simulink model "oms"  (Simulink 6.5)
settings: Solver=ode45  StartTime=0.0  StopTime=10.0  RelTol=1e-3
libraries: cdsFilt x32, cdsEpicsOut x11, cdsMatrix x4, dac x1, simulink x1, cdsSwitch x1, cdsWD x1, cdsParameters x1
(part 2 of 2)

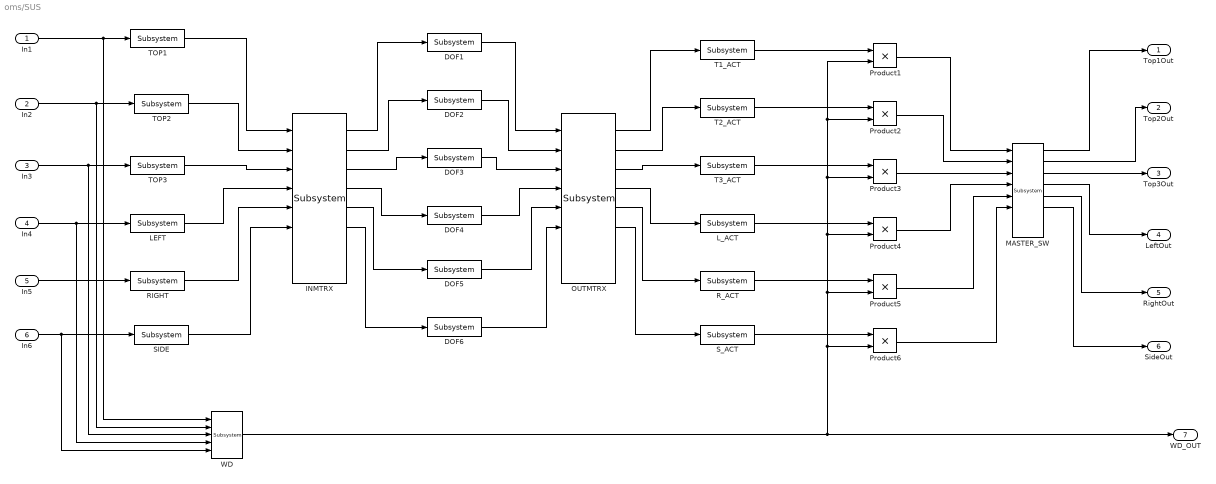
== system oms/SUS ==
  In1 : Inport
  In2 : Inport  Port=2
  In3 : Inport  Port=3
  In4 : Inport  Port=4
  In5 : Inport  Port=5
  In6 : Inport  Port=6
  DOF1 : cdsFilt/Subsystem  Tag=cdsFilt  Description=|  SystemSampleTime=-1
      | Purpose:                                                                                                                                                                                                                                  
      | Standard CDS IIR filter module.                                                                                                                                                                                                           
      |                                                                                                                                                                                                                                           
      | Operation:                                                                                                                                                                                                                                
      | Consists of 10 second order section IIR filters, plus a ramped gain stage. In FE code, also provides pre-defined test points and excitation channel inputs. The filter coefficients are defined in the LIGO system using the 'foton' tool.
      |                                                                                                                                                                                                                                           
      | Usage:                                                                                                                                                                                                                                    
      | Name the part with the desired filter module name.
      settings: AttributesFormatString=%<Tag>
  DOF2 : cdsFilt/Subsystem  Tag=cdsFilt  Description=|  SystemSampleTime=-1
      | Purpose:                                                                                                                                                                                                                                  
      | Standard CDS IIR filter module.                                                                                                                                                                                                           
      |                                                                                                                                                                                                                                           
      | Operation:                                                                                                                                                                                                                                
      | Consists of 10 second order section IIR filters, plus a ramped gain stage. In FE code, also provides pre-defined test points and excitation channel inputs. The filter coefficients are defined in the LIGO system using the 'foton' tool.
      |                                                                                                                                                                                                                                           
      | Usage:                                                                                                                                                                                                                                    
      | Name the part with the desired filter module name.
      settings: AttributesFormatString=%<Tag>
  DOF3 : cdsFilt/Subsystem  Tag=cdsFilt  Description=|  SystemSampleTime=-1
      | Purpose:                                                                                                                                                                                                                                  
      | Standard CDS IIR filter module.                                                                                                                                                                                                           
      |                                                                                                                                                                                                                                           
      | Operation:                                                                                                                                                                                                                                
      | Consists of 10 second order section IIR filters, plus a ramped gain stage. In FE code, also provides pre-defined test points and excitation channel inputs. The filter coefficients are defined in the LIGO system using the 'foton' tool.
      |                                                                                                                                                                                                                                           
      | Usage:                                                                                                                                                                                                                                    
      | Name the part with the desired filter module name.
      settings: AttributesFormatString=%<Tag>
  DOF4 : cdsFilt/Subsystem  Tag=cdsFilt  Description=|  SystemSampleTime=-1
      | Purpose:                                                                                                                                                                                                                                  
      | Standard CDS IIR filter module.                                                                                                                                                                                                           
      |                                                                                                                                                                                                                                           
      | Operation:                                                                                                                                                                                                                                
      | Consists of 10 second order section IIR filters, plus a ramped gain stage. In FE code, also provides pre-defined test points and excitation channel inputs. The filter coefficients are defined in the LIGO system using the 'foton' tool.
      |                                                                                                                                                                                                                                           
      | Usage:                                                                                                                                                                                                                                    
      | Name the part with the desired filter module name.
      settings: AttributesFormatString=%<Tag>
  DOF5 : cdsFilt/Subsystem  Tag=cdsFilt  Description=|  SystemSampleTime=-1
      | Purpose:                                                                                                                                                                                                                                  
      | Standard CDS IIR filter module.                                                                                                                                                                                                           
      |                                                                                                                                                                                                                                           
      | Operation:                                                                                                                                                                                                                                
      | Consists of 10 second order section IIR filters, plus a ramped gain stage. In FE code, also provides pre-defined test points and excitation channel inputs. The filter coefficients are defined in the LIGO system using the 'foton' tool.
      |                                                                                                                                                                                                                                           
      | Usage:                                                                                                                                                                                                                                    
      | Name the part with the desired filter module name.
      settings: AttributesFormatString=%<Tag>
  DOF6 : cdsFilt/Subsystem  Tag=cdsFilt  Description=|  SystemSampleTime=-1
      | Purpose:                                                                                                                                                                                                                                  
      | Standard CDS IIR filter module.                                                                                                                                                                                                           
      |                                                                                                                                                                                                                                           
      | Operation:                                                                                                                                                                                                                                
      | Consists of 10 second order section IIR filters, plus a ramped gain stage. In FE code, also provides pre-defined test points and excitation channel inputs. The filter coefficients are defined in the LIGO system using the 'foton' tool.
      |                                                                                                                                                                                                                                           
      | Usage:                                                                                                                                                                                                                                    
      | Name the part with the desired filter module name.
      settings: AttributesFormatString=%<Tag>
  INMTRX : cdsMatrix/Subsystem  Tag=Matrix  Description=|  SystemSampleTime=-1
      | Purpose:                                                                 
      | Provide a matrix multiplication function for up to 8 input and 8 outputs.
      settings: AttributesFormatString=%<Tag>
  LEFT : cdsFilt/Subsystem  Tag=cdsFilt  Description=|  SystemSampleTime=-1
      | Purpose:                                                                                                                                                                                                                                  
      | Standard CDS IIR filter module.                                                                                                                                                                                                           
      |                                                                                                                                                                                                                                           
      | Operation:                                                                                                                                                                                                                                
      | Consists of 10 second order section IIR filters, plus a ramped gain stage. In FE code, also provides pre-defined test points and excitation channel inputs. The filter coefficients are defined in the LIGO system using the 'foton' tool.
      |                                                                                                                                                                                                                                           
      | Usage:                                                                                                                                                                                                                                    
      | Name the part with the desired filter module name.
      settings: AttributesFormatString=%<Tag>
  L_ACT : cdsFilt/Subsystem  Tag=cdsFilt  Description=|  SystemSampleTime=-1
      | Purpose:                                                                                                                                                                                                                                  
      | Standard CDS IIR filter module.                                                                                                                                                                                                           
      |                                                                                                                                                                                                                                           
      | Operation:                                                                                                                                                                                                                                
      | Consists of 10 second order section IIR filters, plus a ramped gain stage. In FE code, also provides pre-defined test points and excitation channel inputs. The filter coefficients are defined in the LIGO system using the 'foton' tool.
      |                                                                                                                                                                                                                                           
      | Usage:                                                                                                                                                                                                                                    
      | Name the part with the desired filter module name.
      settings: AttributesFormatString=%<Tag>
  MASTER_SW : cdsSwitch/Subsystem  SystemSampleTime=-1
  OUTMTRX : cdsMatrix/Subsystem  Tag=Matrix  Description=|  SystemSampleTime=-1
      | Purpose:                                                                 
      | Provide a matrix multiplication function for up to 8 input and 8 outputs.
      settings: AttributesFormatString=%<Tag>
  Product{1..6} (6 alike) : Product  RndMeth=Zero
  RIGHT : cdsFilt/Subsystem  Tag=cdsFilt  Description=|  SystemSampleTime=-1
      | Purpose:                                                                                                                                                                                                                                  
      | Standard CDS IIR filter module.                                                                                                                                                                                                           
      |                                                                                                                                                                                                                                           
      | Operation:                                                                                                                                                                                                                                
      | Consists of 10 second order section IIR filters, plus a ramped gain stage. In FE code, also provides pre-defined test points and excitation channel inputs. The filter coefficients are defined in the LIGO system using the 'foton' tool.
      |                                                                                                                                                                                                                                           
      | Usage:                                                                                                                                                                                                                                    
      | Name the part with the desired filter module name.
      settings: AttributesFormatString=%<Tag>
  R_ACT : cdsFilt/Subsystem  Tag=cdsFilt  Description=|  SystemSampleTime=-1
      | Purpose:                                                                                                                                                                                                                                  
      | Standard CDS IIR filter module.                                                                                                                                                                                                           
      |                                                                                                                                                                                                                                           
      | Operation:                                                                                                                                                                                                                                
      | Consists of 10 second order section IIR filters, plus a ramped gain stage. In FE code, also provides pre-defined test points and excitation channel inputs. The filter coefficients are defined in the LIGO system using the 'foton' tool.
      |                                                                                                                                                                                                                                           
      | Usage:                                                                                                                                                                                                                                    
      | Name the part with the desired filter module name.
      settings: AttributesFormatString=%<Tag>
  SIDE : cdsFilt/Subsystem  Tag=cdsFilt  Description=|  SystemSampleTime=-1
      | Purpose:                                                                                                                                                                                                                                  
      | Standard CDS IIR filter module.                                                                                                                                                                                                           
      |                                                                                                                                                                                                                                           
      | Operation:                                                                                                                                                                                                                                
      | Consists of 10 second order section IIR filters, plus a ramped gain stage. In FE code, also provides pre-defined test points and excitation channel inputs. The filter coefficients are defined in the LIGO system using the 'foton' tool.
      |                                                                                                                                                                                                                                           
      | Usage:                                                                                                                                                                                                                                    
      | Name the part with the desired filter module name.
      settings: AttributesFormatString=%<Tag>
  S_ACT : cdsFilt/Subsystem  Tag=cdsFilt  Description=|  SystemSampleTime=-1
      | Purpose:                                                                                                                                                                                                                                  
      | Standard CDS IIR filter module.                                                                                                                                                                                                           
      |                                                                                                                                                                                                                                           
      | Operation:                                                                                                                                                                                                                                
      | Consists of 10 second order section IIR filters, plus a ramped gain stage. In FE code, also provides pre-defined test points and excitation channel inputs. The filter coefficients are defined in the LIGO system using the 'foton' tool.
      |                                                                                                                                                                                                                                           
      | Usage:                                                                                                                                                                                                                                    
      | Name the part with the desired filter module name.
      settings: AttributesFormatString=%<Tag>
  T1_ACT : cdsFilt/Subsystem  Tag=cdsFilt  Description=|  SystemSampleTime=-1
      | Purpose:                                                                                                                                                                                                                                  
      | Standard CDS IIR filter module.                                                                                                                                                                                                           
      |                                                                                                                                                                                                                                           
      | Operation:                                                                                                                                                                                                                                
      | Consists of 10 second order section IIR filters, plus a ramped gain stage. In FE code, also provides pre-defined test points and excitation channel inputs. The filter coefficients are defined in the LIGO system using the 'foton' tool.
      |                                                                                                                                                                                                                                           
      | Usage:                                                                                                                                                                                                                                    
      | Name the part with the desired filter module name.
      settings: AttributesFormatString=%<Tag>
  T2_ACT : cdsFilt/Subsystem  Tag=cdsFilt  Description=|  SystemSampleTime=-1
      | Purpose:                                                                                                                                                                                                                                  
      | Standard CDS IIR filter module.                                                                                                                                                                                                           
      |                                                                                                                                                                                                                                           
      | Operation:                                                                                                                                                                                                                                
      | Consists of 10 second order section IIR filters, plus a ramped gain stage. In FE code, also provides pre-defined test points and excitation channel inputs. The filter coefficients are defined in the LIGO system using the 'foton' tool.
      |                                                                                                                                                                                                                                           
      | Usage:                                                                                                                                                                                                                                    
      | Name the part with the desired filter module name.
      settings: AttributesFormatString=%<Tag>
  T3_ACT : cdsFilt/Subsystem  Tag=cdsFilt  Description=|  SystemSampleTime=-1
      | Purpose:                                                                                                                                                                                                                                  
      | Standard CDS IIR filter module.                                                                                                                                                                                                           
      |                                                                                                                                                                                                                                           
      | Operation:                                                                                                                                                                                                                                
      | Consists of 10 second order section IIR filters, plus a ramped gain stage. In FE code, also provides pre-defined test points and excitation channel inputs. The filter coefficients are defined in the LIGO system using the 'foton' tool.
      |                                                                                                                                                                                                                                           
      | Usage:                                                                                                                                                                                                                                    
      | Name the part with the desired filter module name.
      settings: AttributesFormatString=%<Tag>
  TOP1 : cdsFilt/Subsystem  Tag=cdsFilt  Description=|  SystemSampleTime=-1
      | Purpose:                                                                                                                                                                                                                                  
      | Standard CDS IIR filter module.                                                                                                                                                                                                           
      |                                                                                                                                                                                                                                           
      | Operation:                                                                                                                                                                                                                                
      | Consists of 10 second order section IIR filters, plus a ramped gain stage. In FE code, also provides pre-defined test points and excitation channel inputs. The filter coefficients are defined in the LIGO system using the 'foton' tool.
      |                                                                                                                                                                                                                                           
      | Usage:                                                                                                                                                                                                                                    
      | Name the part with the desired filter module name.
      settings: AttributesFormatString=%<Tag>
  TOP2 : cdsFilt/Subsystem  Tag=cdsFilt  Description=|  SystemSampleTime=-1
      | Purpose:                                                                                                                                                                                                                                  
      | Standard CDS IIR filter module.                                                                                                                                                                                                           
      |                                                                                                                                                                                                                                           
      | Operation:                                                                                                                                                                                                                                
      | Consists of 10 second order section IIR filters, plus a ramped gain stage. In FE code, also provides pre-defined test points and excitation channel inputs. The filter coefficients are defined in the LIGO system using the 'foton' tool.
      |                                                                                                                                                                                                                                           
      | Usage:                                                                                                                                                                                                                                    
      | Name the part with the desired filter module name.
      settings: AttributesFormatString=%<Tag>
  TOP3 : cdsFilt/Subsystem  Tag=cdsFilt  Description=|  SystemSampleTime=-1
      | Purpose:                                                                                                                                                                                                                                  
      | Standard CDS IIR filter module.                                                                                                                                                                                                           
      |                                                                                                                                                                                                                                           
      | Operation:                                                                                                                                                                                                                                
      | Consists of 10 second order section IIR filters, plus a ramped gain stage. In FE code, also provides pre-defined test points and excitation channel inputs. The filter coefficients are defined in the LIGO system using the 'foton' tool.
      |                                                                                                                                                                                                                                           
      | Usage:                                                                                                                                                                                                                                    
      | Name the part with the desired filter module name.
      settings: AttributesFormatString=%<Tag>
  WD : cdsWD/Subsystem  SystemSampleTime=-1
  Top1Out : Outport
  Top2Out : Outport  Port=2
  Top3Out : Outport  Port=3
  LeftOut : Outport  Port=4
  RightOut : Outport  Port=5
  SideOut : Outport  Port=6
  WD_OUT : Outport  Port=7
  wires:
  OUTMTRX/6 -> S_ACT/1
  OUTMTRX/5 -> R_ACT/1
  OUTMTRX/4 -> L_ACT/1
  OUTMTRX/3 -> T3_ACT/1
  OUTMTRX/2 -> T2_ACT/1
  OUTMTRX/1 -> T1_ACT/1
  DOF6/1 -> OUTMTRX/6
  DOF5/1 -> OUTMTRX/5
  DOF4/1 -> OUTMTRX/4
  DOF3/1 -> OUTMTRX/3
  DOF2/1 -> OUTMTRX/2
  DOF1/1 -> OUTMTRX/1
  INMTRX/6 -> DOF6/1
  INMTRX/5 -> DOF5/1
  INMTRX/4 -> DOF4/1
  INMTRX/3 -> DOF3/1
  INMTRX/2 -> DOF2/1
  INMTRX/1 -> DOF1/1
  SIDE/1 -> INMTRX/6
  RIGHT/1 -> INMTRX/5
  LEFT/1 -> INMTRX/4
  TOP3/1 -> INMTRX/3
  TOP2/1 -> INMTRX/2
  TOP1/1 -> INMTRX/1
  In1/1 -> WD/1, TOP1/1
  In2/1 -> WD/2, TOP2/1
  In3/1 -> WD/3, TOP3/1
  In4/1 -> WD/4, LEFT/1
  In5/1 -> RIGHT/1
  In6/1 -> WD/5, SIDE/1
  WD/1 -> WD_OUT/1, Product6/2, Product5/2, Product4/2, Product3/2, Product2/2, Product1/2
  T1_ACT/1 -> Product1/1
  T2_ACT/1 -> Product2/1
  T3_ACT/1 -> Product3/1
  L_ACT/1 -> Product4/1
  R_ACT/1 -> Product5/1
  S_ACT/1 -> Product6/1
  Product1/1 -> MASTER_SW/1
  Product2/1 -> MASTER_SW/2
  Product3/1 -> MASTER_SW/3
  Product4/1 -> MASTER_SW/4
  Product5/1 -> MASTER_SW/5
  Product6/1 -> MASTER_SW/6
  MASTER_SW/1 -> Top1Out/1
  MASTER_SW/2 -> Top2Out/1
  MASTER_SW/3 -> Top3Out/1
  MASTER_SW/4 -> LeftOut/1
  MASTER_SW/5 -> RightOut/1
  MASTER_SW/6 -> SideOut/1
